simulink model "sbic_proj_2020a"  (R2020b)
settings: Solver=VariableStepAuto  StartTime=0.0  StopTime=500  RelTol=1e-3
values from neighbouring files (symbols this model uses):
  A = [ -1/(2*T) 0; 0  -1/T]    [main.m]
  B = [1/S 1/S; (C1-C0)/(S*H0) (C2-C0)/(S*H0)]    [main.m]
  C = [1 0; 0 1]    [main.m]
  D = [0 0; 0 0]    [main.m]
libraries: fuzblock x13
settings Model: Creator=tecas  LastModifiedBy=ManuelMaria
settings SolverCC: ZeroCrossAlgorithm=Adaptive
settings DebuggingCC: IgnoredZcDiagnostic=none

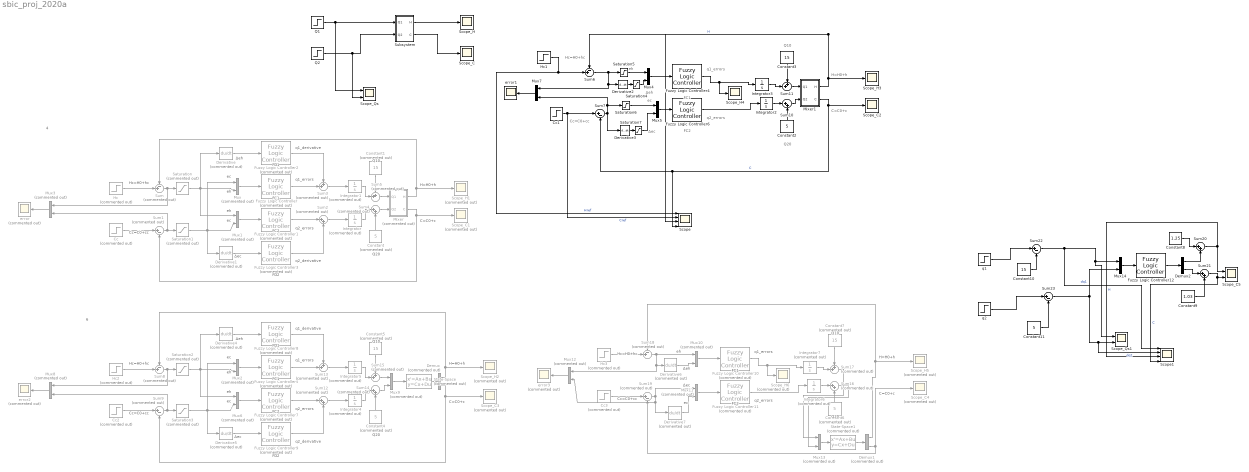
== system sbic_proj_2020a ==
  note: 4
  note: Hc=H0+hc
  note: eh
  note: FC1
  note: Q20
  note: q1_errors
  note: q2_errors
  note: Q10
  note: FC2
  note: FD2
  note: FD1
  note: eh
  note: Δeh
  note: Δec
  note: ec
  note: ec
  note: Cc=C0+cc
  note: H=H0+h
  note: C=C0+c
  note: q2_derivative
  note: q1_derivative
  note: Δeh
  note: Δec
  note: Cc=C0+cc
  note: ec
  note: Hc=H0+hc
  note: eh
  note: FC1
  note: Q20
  note: q1_errors
  note: q2_errors
  note: Q10
  note: C=C0+c
  note: H=H0+h
  note: FC2
  note: FC1
  note: eh
  note: Hc=H0+hc
  note: H=H0+h
  note: Q20
  note: FD2
  note: Q10
  note: Cc=C0+cc
  note: FD1
  note: q1_errors
  note: ec
  note: q2_errors
  note: ec
  note: eh
  note: C=C0+c
  note: FC2
  note: q2_derivative
  note: Δeh
  note: q1_derivative
  note: Δec
  note: H=H0+h
  note: FC1
  note: Q10
  note: eh
  note: Q20
  note: C=C0+c
  note: Δec
  note: Cc=C0+cc
  note: Hc=H0+hc
  note: q2_errors
  note: q1_errors
  note: Δeh
  note: FC2
  note: ec
  note: 6
  Cc : Step  Commented=on  Time=15  Before=1  After=5  SampleTime=0
  Cc1 : Step  Time=15  Before=1  After=3  SampleTime=0
  Cc2 : Step  Commented=on  Time=15  Before=3  After=3  SampleTime=0
  Cc3 : Step  Commented=on  Time=15  After=5  SampleTime=0
  Constant : Constant  Commented=on  Value=5
  Constant1 : Constant  Commented=on  Value=15
  Constant10 : Constant  Value=15
  Constant11 : Constant  Value=5
  Constant2 : Constant  Value=5
  Constant3 : Constant  Value=15
  Constant4 : Constant  Commented=on  Value=5
  Constant5 : Constant  Commented=on  Value=15
  Constant6 : Constant  Commented=on  Value=5
  Constant7 : Constant  Commented=on  Value=15
  Constant8 : Constant  Value=1.25
  Constant9 : Constant  Value=1.03
  Demux : Demux  Commented=on  Outputs=2
  Demux1 : Demux  Commented=on  Outputs=2
  Demux2 : Demux  Outputs=2
  Derivative{,1,4..7} (6 alike) : Derivative  Commented=on
  Derivative2 : Derivative
  Derivative3 : Derivative
  Fuzzy Logic Controller{,1,5,7} (4 alike) : fuzblock/Fuzzy Logic  Controller  Commented=on  FIS=FC2_3  OutputSampleNumber=101  DataType=double  FuzzifiedInputs=off  RuleFiringStrengths=off  RuleOutputs=off  AggregatedOutputs=off  SimulateUsing=Interpreted execution  OutOfRangeInputValueMessage=warning  NoRuleFiredMessage=warning  EmptyOutputFuzzySetMessage=warning
  Fuzzy Logic Controller10 : fuzblock/Fuzzy Logic  Controller  Commented=on  FIS=FC1_ex3  OutputSampleNumber=101  DataType=double  FuzzifiedInputs=off  RuleFiringStrengths=off  RuleOutputs=off  AggregatedOutputs=off  SimulateUsing=Interpreted execution  OutOfRangeInputValueMessage=warning  NoRuleFiredMessage=warning  EmptyOutputFuzzySetMessage=warning
  Fuzzy Logic Controller11 : fuzblock/Fuzzy Logic  Controller  Commented=on  FIS=FC2_ex3  OutputSampleNumber=101  DataType=double  FuzzifiedInputs=off  RuleFiringStrengths=off  RuleOutputs=off  AggregatedOutputs=off  SimulateUsing=Interpreted execution  OutOfRangeInputValueMessage=warning  NoRuleFiredMessage=warning  EmptyOutputFuzzySetMessage=warning
  Fuzzy Logic Controller12 : fuzblock/Fuzzy Logic  Controller  FIS=fuzzy_model  OutputSampleNumber=101  DataType=double  FuzzifiedInputs=off  RuleFiringStrengths=off  RuleOutputs=off  AggregatedOutputs=off  SimulateUsing=Interpreted execution  OutOfRangeInputValueMessage=warning  NoRuleFiredMessage=warning  EmptyOutputFuzzySetMessage=warning
  Fuzzy Logic Controller{2..3,8..9} (4 alike) : fuzblock/Fuzzy Logic  Controller  Commented=on  FIS=FD  OutputSampleNumber=101  DataType=double  FuzzifiedInputs=off  RuleFiringStrengths=off  RuleOutputs=off  AggregatedOutputs=off  SimulateUsing=Interpreted execution  OutOfRangeInputValueMessage=warning  NoRuleFiredMessage=warning  EmptyOutputFuzzySetMessage=warning
  Fuzzy Logic Controller4 : fuzblock/Fuzzy Logic  Controller  FIS=FC1_ex3  OutputSampleNumber=101  DataType=double  FuzzifiedInputs=off  RuleFiringStrengths=off  RuleOutputs=off  AggregatedOutputs=off  SimulateUsing=Interpreted execution  OutOfRangeInputValueMessage=warning  NoRuleFiredMessage=warning  EmptyOutputFuzzySetMessage=warning
  Fuzzy Logic Controller6 : fuzblock/Fuzzy Logic  Controller  FIS=FC2_ex3  OutputSampleNumber=101  DataType=double  FuzzifiedInputs=off  RuleFiringStrengths=off  RuleOutputs=off  AggregatedOutputs=off  SimulateUsing=Interpreted execution  OutOfRangeInputValueMessage=warning  NoRuleFiredMessage=warning  EmptyOutputFuzzySetMessage=warning
  Hc : Step  Commented=on  Time=15  Before=5  After=15  SampleTime=0
  Hc1 : Step  Time=100  Before=1  After=5  SampleTime=0
  Hc2 : Step  Commented=on  Time=15  Before=5  After=15  SampleTime=0
  Hc3 : Step  Commented=on  Time=15  After=5  SampleTime=0
  Integrator{,1,4..5} (4 alike) : Integrator  Commented=on  InitialCondition=0.1
  Integrator2 : Integrator  InitialCondition=0.1
  Integrator3 : Integrator  InitialCondition=0.1
  Integrator6 : Integrator  Commented=on
  Integrator7 : Integrator  Commented=on
  Mixer : Subsystem  Commented=on
  Mixer1 : Subsystem
  Mux{,1..3,6,8..13} (11 alike) : Mux  Commented=on  Inputs=2
  Mux{4..5,7,14} (4 alike) : Mux  Inputs=2
  Q1 : Step  Time=15  Before=15  After=15  SampleTime=0
  Q2 : Step  Time=15  Before=5  After=5  SampleTime=0
  Saturation{,1..3} (4 alike) : Saturate  Commented=on  UpperLimit=1  LowerLimit=-1
  Saturation4 : Saturate  UpperLimit=3  LowerLimit=-3
  Saturation5 : Saturate  UpperLimit=5  LowerLimit=-5
  Saturation6 : Saturate  UpperLimit=3  LowerLimit=-3
  Saturation7 : Saturate  UpperLimit=3  LowerLimit=-3
  Scope : Scope  NumInputPorts=4
  Scope1 : Scope  NumInputPorts=4
  Scope_C : Scope
  Scope_C1 : Scope  Commented=on
  Scope_C2 : Scope
  Scope_C3 : Scope  Commented=on
  Scope_C4 : Scope  Commented=on
  Scope_C5 : Scope  NumInputPorts=2
  Scope_H : Scope
  Scope_H{1..2,5..6} (4 alike) : Scope  Commented=on
  Scope_H3 : Scope
  Scope_H4 : Scope
  Scope_Qs : Scope  NumInputPorts=2
  Scope_Qs1 : Scope  NumInputPorts=2
  State-Space : StateSpace  Commented=on  A=A  B=B  C=C  D=D  InitialCondition=0
  State-Space1 : StateSpace  Commented=on  A=A  B=B  C=C  D=D  InitialCondition=0
  Subsystem : Subsystem
  Sum : Sum  Commented=on  Inputs=-+|
  Sum1 : Sum  Commented=on  Inputs=|+-
  Sum10 : Sum  Inputs=|++
  Sum11 : Sum  Inputs=++|
  Sum{2,4,12,14,16} (5 alike) : Sum  Commented=on  Inputs=|++
  Sum{3,5,13,15,17} (5 alike) : Sum  Commented=on  Inputs=++|
  Sum18 : Sum  Commented=on  Inputs=-+|
  Sum19 : Sum  Commented=on  Inputs=|+-
  Sum20 : Sum  Inputs=|++
  Sum21 : Sum  Inputs=|++
  Sum22 : Sum  Inputs=|+-
  Sum23 : Sum  Inputs=|+-
  Sum6 : Sum  Inputs=-+|
  Sum7 : Sum  Inputs=|+-
  Sum8 : Sum  Commented=on  Inputs=-+|
  Sum9 : Sum  Commented=on  Inputs=|+-
  error : Scope  Commented=on
  error1 : Scope
  error2 : Scope  Commented=on
  error3 : Scope  Commented=on
  q1 : Step  Time=100  Before=15  After=18  SampleTime=0
  q2 : Step  Time=100  Before=5  After=6.5  SampleTime=0
  wires:
  Q1/1 -> Subsystem/1(Q1), Scope_Qs/1
  Q2/1 -> Scope_Qs/2, Subsystem/2(Q2)
  Subsystem/1(H) -> Scope_H/1
  Subsystem/2(C) -> Scope_C/1
  Mixer/2(C) -> Sum1/2, Scope_C1/1
  Mixer/1(H) -> Sum/1, Scope_H1/1
  Mux/1 -> Fuzzy Logic Controller/1
  Mux1/1 -> Fuzzy Logic Controller1/1
  Hc/1 -> Sum/2
  Cc/1 -> Sum1/1
  Sum1/1 -> Mux3/2, Saturation1/1
  Fuzzy Logic Controller1/1 -> Sum2/1
  Sum2/1 -> Integrator/1
  Fuzzy Logic Controller/1 -> Sum3/2
  Sum3/1 -> Integrator1/1
  Integrator/1 -> Sum4/1
  Sum4/1 -> Mixer/2(Q2)
  Integrator1/1 -> Sum5/2
  Sum5/1 -> Mixer/1(Q1)
  Constant/1 -> Sum4/2
  Constant1/1 -> Sum5/1
  Derivative1/1 -> Fuzzy Logic Controller3/1
  Derivative/1 -> Fuzzy Logic Controller2/1
  Fuzzy Logic Controller2/1 -> Sum3/1
  Fuzzy Logic Controller3/1 -> Sum2/2
  Mux3/1 -> error/1
  Sum/1 -> Mux3/1, Saturation/1
  Sum7/1 -> Saturation6/1, Mux7/2, Derivative3/1
  Fuzzy Logic Controller4/1 -> Scope_H4/1, Integrator3/1
  Hc1/1 -> Sum6/2, Scope/1  "Href"
  Sum11/1 -> Mixer1/1(Q1)
  Integrator3/1 -> Sum11/2
  Integrator2/1 -> Sum10/1
  Constant3/1 -> Sum11/1
  Mux7/1 -> error1/1
  Cc1/1 -> Scope/2, Sum7/1  "Cref"
  Mixer1/1(H) -> Scope/3, Sum6/1, Scope_H3/1  "H"
  Mux4/1 -> Fuzzy Logic Controller4/1
  Mux5/1 -> Fuzzy Logic Controller6/1
  Mixer1/2(C) -> Scope_C2/1, Scope/4, Sum7/2  "C"
  Fuzzy Logic Controller6/1 -> Integrator2/1
  Constant2/1 -> Sum10/2
  Sum10/1 -> Mixer1/2(Q2)
  Saturation/1 -> Mux1/1, Mux/2, Derivative/1
  Saturation1/1 -> Mux/1, Mux1/2, Derivative1/1
  Saturation3/1 -> Mux2/1, Mux6/2, Derivative5/1
  Mux2/1 -> Fuzzy Logic Controller5/1
  Sum15/1 -> Mux9/1
  Saturation2/1 -> Mux6/1, Mux2/2, Derivative4/1
  Hc2/1 -> Sum8/2
  Derivative4/1 -> Fuzzy Logic Controller8/1
  Constant5/1 -> Sum15/1
  Constant4/1 -> Sum14/2
  Derivative5/1 -> Fuzzy Logic Controller9/1
  Fuzzy Logic Controller9/1 -> Sum12/2
  Mux8/1 -> error2/1
  Fuzzy Logic Controller7/1 -> Sum12/1
  Sum12/1 -> Integrator4/1
  Mux6/1 -> Fuzzy Logic Controller7/1
  Integrator4/1 -> Sum14/1
  Integrator5/1 -> Sum15/2
  Demux/2 -> Sum9/2, Scope_C3/1
  Sum13/1 -> Integrator5/1
  Sum9/1 -> Mux8/2, Saturation3/1
  Fuzzy Logic Controller5/1 -> Sum13/2
  Cc2/1 -> Sum9/1
  Fuzzy Logic Controller8/1 -> Sum13/1
  Demux/1 -> Sum8/1, Scope_H2/1
  Sum8/1 -> Mux8/1, Saturation2/1
  Mux9/1 -> State-Space/1
  Sum14/1 -> Mux9/2
  State-Space/1 -> Demux/1
  Constant7/1 -> Sum17/1
  Constant6/1 -> Sum16/2
  Demux1/2 -> Scope_C4/1, Sum19/2
  Derivative6/1 -> Mux10/2
  Integrator7/1 -> Sum17/2
  Fuzzy Logic Controller11/1 -> Integrator6/1
  Mux11/1 -> Fuzzy Logic Controller11/1
  Cc3/1 -> Sum19/1
  Mux12/1 -> error3/1
  Mux10/1 -> Fuzzy Logic Controller10/1
  Hc3/1 -> Sum18/2
  Demux1/1 -> Sum18/1, Scope_H5/1
  Derivative7/1 -> Mux11/2
  Fuzzy Logic Controller10/1 -> Scope_H6/1, Integrator7/1
  Sum19/1 -> Mux12/2, Derivative7/1, Mux11/1
  Integrator6/1 -> Sum16/1
  Sum18/1 -> Mux10/1, Mux12/1, Derivative6/1
  State-Space1/1 -> Demux1/1
  Sum17/1 -> Mux13/1
  Sum16/1 -> Mux13/2
  Mux13/1 -> State-Space1/1
  Sum6/1 -> Saturation5/1, Derivative2/1, Mux7/1
  Derivative2/1 -> Saturation4/1
  Saturation4/1 -> Mux4/2
  Saturation5/1 -> Mux4/1
  Saturation6/1 -> Mux5/1
  Derivative3/1 -> Saturation7/1
  Saturation7/1 -> Mux5/2
  q1/1 -> Sum22/1
  q2/1 -> Sum23/1
  Mux14/1 -> Fuzzy Logic Controller12/1
  Fuzzy Logic Controller12/1 -> Demux2/1
  Constant8/1 -> Sum20/1
  Demux2/1 -> Sum20/2
  Sum20/1 -> Scope_C5/1, Scope1/3  "H"
  Demux2/2 -> Sum21/1
  Constant9/1 -> Sum21/2
  Sum23/1 -> Mux14/2, Scope1/2, Scope_Qs1/2  "dq2"
  Constant10/1 -> Sum22/2
  Constant11/1 -> Sum23/2
  Sum21/1 -> Scope1/4, Scope_C5/2  "C"
  Sum22/1 -> Scope1/1, Scope_Qs1/1, Mux14/1  "dq1"

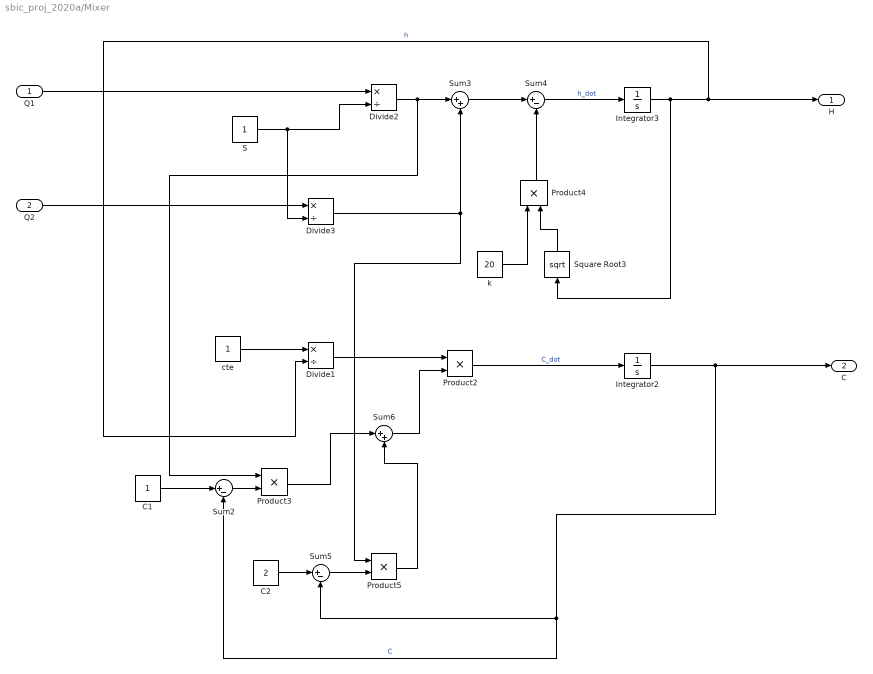
== system sbic_proj_2020a/Mixer ==
  Q1 : Inport
  Q2 : Inport  Port=2
  C1 : Constant
  C2 : Constant  Value=2
  Divide1 : Product  Inputs=*/
  Divide2 : Product  Inputs=*/
  Divide3 : Product  Inputs=*/
  Integrator2 : Integrator  InitialCondition=1.25
  Integrator3 : Integrator  InitialCondition=1
  Product{2..5} (4 alike) : Product
  S : Constant
  Square Root3 : Sqrt  SaturateOnIntegerOverflow=on
  Sum2 : Sum  Inputs=|+-
  Sum3 : Sum  Inputs=|++
  Sum4 : Sum  Inputs=|+-
  Sum5 : Sum  Inputs=|+-
  Sum6 : Sum  Inputs=|++
  cte : Constant
  k : Constant  Value=20
  H : Outport
  C : Outport  Port=2
  wires:
  C1/1 -> Sum2/1
  C2/1 -> Sum5/1
  Product4/1 -> Sum4/2
  Product2/1 -> Integrator2/1  "C_dot"
  Integrator2/1 -> C/1, Sum5/2, Sum2/2  "C"
  S/1 -> Divide2/2, Divide3/2
  Integrator3/1 -> H/1, Divide1/2, Square Root3/1  "h"
  Sum3/1 -> Sum4/1
  Sum2/1 -> Product3/2
  Product5/1 -> Sum6/2
  Product3/1 -> Sum6/1
  Divide3/1 -> Product5/1, Sum3/2
  Sum5/1 -> Product5/2
  Sum4/1 -> Integrator3/1  "h_dot"
  cte/1 -> Divide1/1
  Divide2/1 -> Product3/1, Sum3/1
  Square Root3/1 -> Product4/2
  Q2/1 -> Divide3/1
  Q1/1 -> Divide2/1
  Divide1/1 -> Product2/1
  Sum6/1 -> Product2/2
  k/1 -> Product4/1

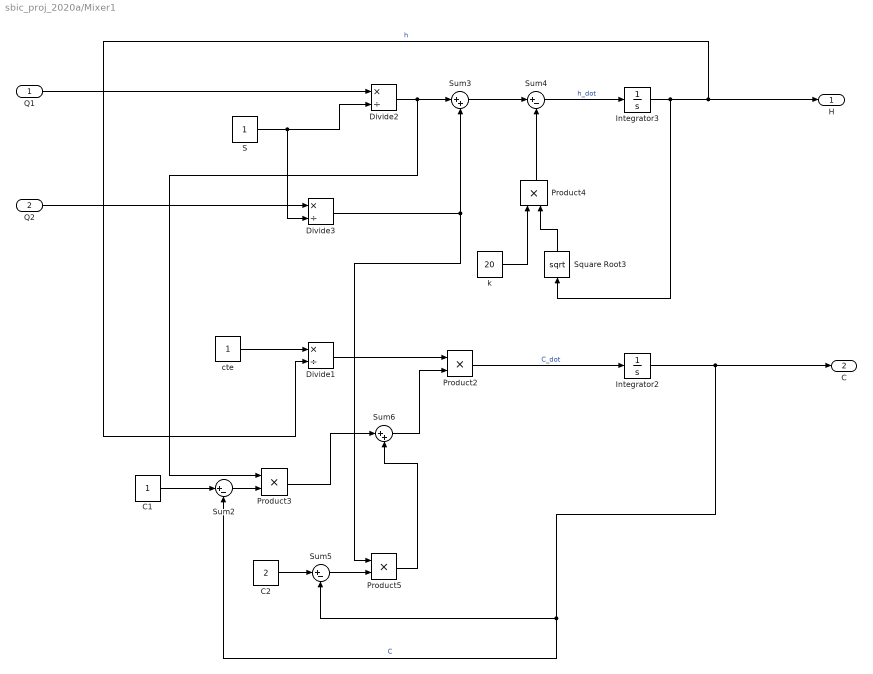
== system sbic_proj_2020a/Mixer1 ==
  Q1 : Inport
  Q2 : Inport  Port=2
  C1 : Constant
  C2 : Constant  Value=2
  Divide1 : Product  Inputs=*/
  Divide2 : Product  Inputs=*/
  Divide3 : Product  Inputs=*/
  Integrator2 : Integrator  InitialCondition=1.25
  Integrator3 : Integrator  InitialCondition=1
  Product{2..5} (4 alike) : Product
  S : Constant
  Square Root3 : Sqrt  SaturateOnIntegerOverflow=on
  Sum2 : Sum  Inputs=|+-
  Sum3 : Sum  Inputs=|++
  Sum4 : Sum  Inputs=|+-
  Sum5 : Sum  Inputs=|+-
  Sum6 : Sum  Inputs=|++
  cte : Constant
  k : Constant  Value=20
  H : Outport
  C : Outport  Port=2
  wires:
  C1/1 -> Sum2/1
  C2/1 -> Sum5/1
  Product4/1 -> Sum4/2
  Product2/1 -> Integrator2/1  "C_dot"
  Integrator2/1 -> C/1, Sum5/2, Sum2/2  "C"
  S/1 -> Divide2/2, Divide3/2
  Integrator3/1 -> H/1, Divide1/2, Square Root3/1  "h"
  Sum3/1 -> Sum4/1
  Sum2/1 -> Product3/2
  Product5/1 -> Sum6/2
  Product3/1 -> Sum6/1
  Divide3/1 -> Product5/1, Sum3/2
  Sum5/1 -> Product5/2
  Sum4/1 -> Integrator3/1  "h_dot"
  cte/1 -> Divide1/1
  Divide2/1 -> Product3/1, Sum3/1
  Square Root3/1 -> Product4/2
  Q2/1 -> Divide3/1
  Q1/1 -> Divide2/1
  Divide1/1 -> Product2/1
  Sum6/1 -> Product2/2
  k/1 -> Product4/1

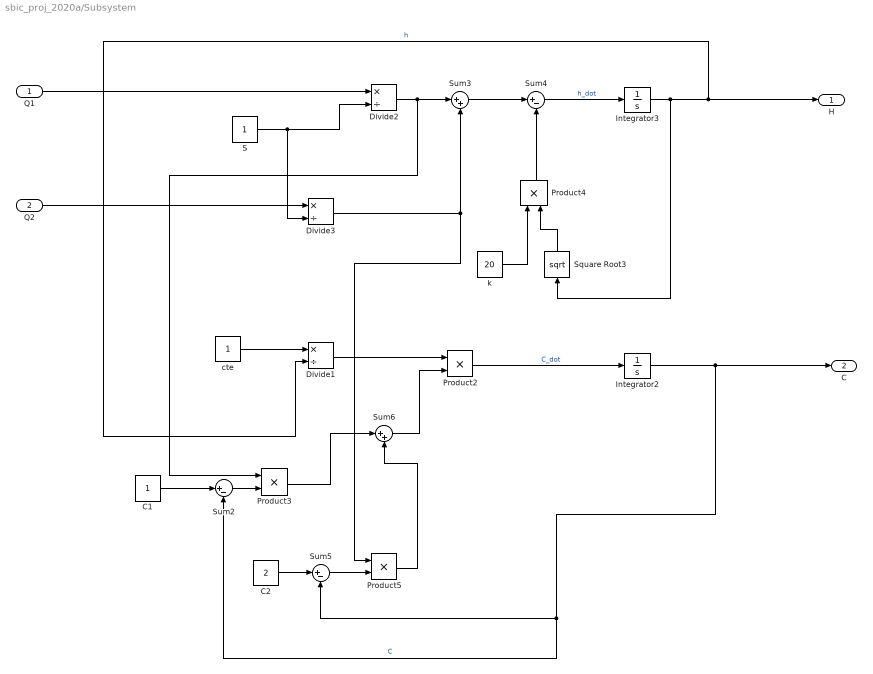
== system sbic_proj_2020a/Subsystem ==
  Q1 : Inport
  Q2 : Inport  Port=2
  C1 : Constant
  C2 : Constant  Value=2
  Divide1 : Product  Inputs=*/
  Divide2 : Product  Inputs=*/
  Divide3 : Product  Inputs=*/
  Integrator2 : Integrator  InitialCondition=1.25
  Integrator3 : Integrator  InitialCondition=1
  Product{2..5} (4 alike) : Product
  S : Constant
  Square Root3 : Sqrt  SaturateOnIntegerOverflow=on
  Sum2 : Sum  Inputs=|+-
  Sum3 : Sum  Inputs=|++
  Sum4 : Sum  Inputs=|+-
  Sum5 : Sum  Inputs=|+-
  Sum6 : Sum  Inputs=|++
  cte : Constant
  k : Constant  Value=20
  H : Outport
  C : Outport  Port=2
  wires:
  C1/1 -> Sum2/1
  C2/1 -> Sum5/1
  Product4/1 -> Sum4/2
  Product2/1 -> Integrator2/1  "C_dot"
  Integrator2/1 -> C/1, Sum5/2, Sum2/2  "C"
  S/1 -> Divide2/2, Divide3/2
  Integrator3/1 -> H/1, Divide1/2, Square Root3/1  "h"
  Sum3/1 -> Sum4/1
  Sum2/1 -> Product3/2
  Product5/1 -> Sum6/2
  Product3/1 -> Sum6/1
  Divide3/1 -> Product5/1, Sum3/2
  Sum5/1 -> Product5/2
  Sum4/1 -> Integrator3/1  "h_dot"
  cte/1 -> Divide1/1
  Divide2/1 -> Product3/1, Sum3/1
  Square Root3/1 -> Product4/2
  Q2/1 -> Divide3/1
  Q1/1 -> Divide2/1
  Divide1/1 -> Product2/1
  Sum6/1 -> Product2/2
  k/1 -> Product4/1
